simulink model "test_mdl_NI"  (R2018a)
settings: Solver=VariableStepAuto  StartTime=0.0  StopTime=10.0  RelTol=1e-3
(part 2 of 24)

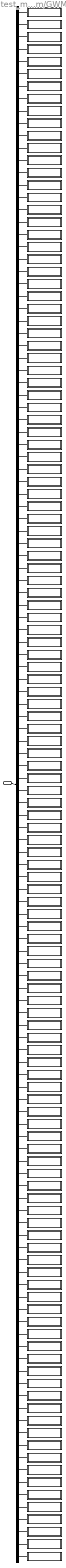
== system test_mdl_NI/Subsystem/GWM ==
  in_port : Inport
  AC_Compressor_Data_FD1_Ox411 : Subsystem
  APIMGPS_Data_Nav_1_FD1_Ox462 : Subsystem
  APIMGPS_Data_Nav_2_FD1_Ox463 : Subsystem
  APIMGPS_Data_Nav_3_FD1_Ox464 : Subsystem
  APIM_Data_FD1_Ox32B : Subsystem
  APIM_Request_Signals_1_FD1_Ox227 : Subsystem
  APIM_Request_Signals_5_FD1_Ox211 : Subsystem
  APIM_Request_Signals_FD1_Ox105 : Subsystem
  APIM_Send_Signals1_FD1_Ox3F1 : Subsystem
  APIM_Send_Signals_2_FD1_Ox215 : Subsystem
  Accel_Data_FD1_Ox92 : Subsystem
  ActiveFrontStrg_Stat2_FD1_Ox8A : Subsystem
  ActiveFrontStrg_Stat_FD1_Ox89 : Subsystem
  Adaptive_Headlamp_Stat_Ox334 : Subsystem
  AllTerrainControlData_FD1_Ox461 : Subsystem
  All_Terrain_Data_FD1_Ox481 : Subsystem
  BCMC_Data_FD1_Ox36F : Subsystem
  BCM_Lamp_Stat_FD1_Ox3C3 : Subsystem
  BattRgenLo_1_FD1_Ox361 : Subsystem
  BattRgenLo_2_FD1_Ox362 : Subsystem
  BattRgenLo_3_FD1_Ox363 : Subsystem
  BattRgenLo_4_FD1_Ox364 : Subsystem
  Battery_Mgmt_24V_FD1_Ox42E : Subsystem
  Battery_Mgmt_2_FD1_Ox42C : Subsystem
  Battery_Mgmt_3_FD1_Ox43C : Subsystem
  Battery_Mgmt_4_FD1_Ox42B : Subsystem
  Battery_Traction_1_FD1_Ox7A : Subsystem
  Battery_Traction_3_FD1_Ox24B : Subsystem
  Battery_Traction_4_FD1_Ox24C : Subsystem
  Battery_Traction_5_FD1_Ox24D : Subsystem
  Battery_Traction_6_FD1_Ox458 : Subsystem
  BodyInfo_3_FD1_Ox3B3 : Subsystem
  Body_Info_10_FD1_Ox3BA : Subsystem
  Body_Info_4_FD1_Ox242 : Subsystem
  Body_Info_6_FD1_Ox38D : Subsystem
  Body_Info_8_FD1_Ox3B9 : Subsystem
  Body_Info_9_FD1_Ox3A3 : Subsystem
  Climate_Cntrl_Data_2_FD1_Ox35E : Subsystem
  Climate_Control_Data_FD1_Ox41A : Subsystem
  Cluster_HEV_Data8_FD1_Ox317 : Subsystem
  Cluster_Info1_FD1_Ox430 : Subsystem
  Cluster_Info_3_FD1_Ox434 : Subsystem
  Cluster_Lighting_Rq_FD1_Ox3C8 : Subsystem
  Compressor_Req_FD1_Ox326 : Subsystem
  CruiseCtrl_Strg_Data_FD1_Ox8B : Subsystem
  DCACA_Data1_FD1_Ox39A : Subsystem
  DCACA_Data2_FD1_Ox39B : Subsystem
  DCACA_Data3_FD1_Ox39C : Subsystem
  DTE_ECGtoHPCM_Ox338 : Subsystem
  Driver_Dr_Stat_FD1_Ox332 : Subsystem
  Dsp_Request_Signals11_FD1_Ox192 : Subsystem
  ECG_Data2_FD1_Ox488 : Subsystem
  ECG_Data3_FD1_Ox375 : Subsystem
  ECG_Data4_FD1_Ox226 : Subsystem
  ECG_Data_FD1_Ox32A : Subsystem
  ElecHorizon_Data1_FD1_Ox22E : Subsystem
  ElecHorizon_Data2_FD1_Ox22F : Subsystem
  FourByFourSwitchData_FD1_Ox460 : Subsystem
  GGCC_Config_Mgmt_ID_1_FD1_Ox40A : Subsystem
  GWM_AutoSar_NetMgmt_FD1_Ox59E : Subsystem
  Gear_Shift_by_Wire_2_FD1_Ox168 : Subsystem
  Gear_Shift_by_Wire_FD1_Ox5A : Subsystem
  GlobalClock_Data_FD1_Ox84 : Subsystem
  Global_PATS_Cntrl_Info_FD1_Ox41 : Subsystem
  Global_PATS_Ctrl_Info2_FD1_Ox42 : Subsystem
  HeadUpDisplayReq_FD1_Ox18B : Subsystem
  IPC_Infotainment_FD1_Ox225 : Subsystem
  IPC_Send_Signals_2_FD1_Ox318 : Subsystem
  LocationServices_3_FD1_Ox21E : Subsystem
  LocationServices_Data1_FD1_Ox47E : Subsystem
  Locking_Systems_2_FD1_Ox331 : Subsystem
  MasterReset_HS3_ECGDat_FD1_Ox233 : Subsystem
  Mc_Send_Signals_2_FD1_Ox2FD : Subsystem
  OTAFuncGWM_ECG_FD1_Ox1B9FFCD8 : Subsystem
  OTAPhysGWM_ECGtoABS_Ox1B90A0D8 : Subsystem
  OTAPhysGWM_ECGtoCCM_Ox1B9054D8 : Subsystem
  OTAPhysGWM_ECGtoIPMA_Ox1B9084D8 : Subsystem
  OTAPhysGWM_ECGtoPCM_Ox1B9040D8 : Subsystem
  OTAPhysGWM_ECGtoSOBDMC_FD1_Ox1B9044D8 : Subsystem
  OTAPhysGWM_ECGtoSODCMC_Ox1B9114D8 : Subsystem
  OTAPhysGWM_ECGtoSODCMD_Ox1B9118D8 : Subsystem
  OTAPhysGWM_ECGtoSODL_Ox1B9188D8 : Subsystem
  OTAPhysGWM_ECGtoSODR_Ox1B918CD8 : Subsystem
  OffBrdChrg_Signals2_Ox27F : Subsystem
  OffBrdChrg_Signals_Ox212 : Subsystem
  PARSEDFuncGWM_ECG_FD1_Ox1BAFFCD8 : Subsystem
  PARSEDPhysGWM_ECGtoABS_Ox1BA0A0D8 : Subsystem
  PARSEDPhysGWM_ECGtoCCM_Ox1BA054D8 : Subsystem
  PARSEDPhysGWM_ECGtoIPMA_Ox1BA084D8 : Subsystem
  PARSEDPhysGWM_ECGtoPCM_Ox1BA040D8 : Subsystem
  PARSEDPhysGWM_ECGtoSODCMC_Ox1BA114D8 : Subsystem
  PARSEDPhysGWM_ECGtoSODCMD_Ox1BA118D8 : Subsystem
  PARSEDPhysGWM_ECGtoSODL_Ox1BA188D8 : Subsystem
  PARSEDPhysGWM_ECGtoSODR_Ox1BA18CD8 : Subsystem
  PARSEDPhysGWMtoSOBDMC_FD1_Ox1BA044D8 : Subsystem
  PARSEDPushFcGWM_ECGtoABS_Ox1BB0A0D8 : Subsystem
  PARSEDPushFcGWM_ECGtoPCM_Ox1BB040D8 : Subsystem
  PHEV_Battery_Data1_FD1_Ox2E4 : Subsystem
  ParkAid_Aud_Warn_CmdM_FD1_Ox30A : Subsystem
  Pass_Dr_Stat_FD1_Ox333 : Subsystem
  Personality_APIM_Data_FD1_Ox3E2 : Subsystem
  Personality_BCM2_Data_FD1_Ox3EB : Subsystem
  Personality_Data_FD1_Ox3E0 : Subsystem
  PowerDistData_2_FD1_Ox36A : Subsystem
  PowerDist_Data1_FD1_Ox390 : Subsystem
  Power_Liftgate_Stat_FD1_Ox313 : Subsystem
  RCMSerialNumber_FD1_Ox454 : Subsystem
  RCMStatusMessage2_FD1_Ox4C : Subsystem
  SmartChargingData_ECG_1_Ox306 : Subsystem
  SmartChargingData_ECG_2_Ox307 : Subsystem
  SmartChargingData_ECG_3_Ox308 : Subsystem
  Steering_Data_FD1_Ox83 : Subsystem
  Steering_Wheel_Data2_FD1_Ox81 : Subsystem
  TCU_Send_Signals_FD1_Ox28B : Subsystem
  TesterPhysicalReqVDM_FD1_Ox721 : Subsystem
  TesterPhysicalResGWM_FD1_Ox71E : Subsystem
  Tire_Pressure_Data_FD1_Ox3B5 : Subsystem
  TrailerAid_Data3_FD1_Ox45C : Subsystem
  TrailerAid_Data_FD1_Ox45A : Subsystem
  TrailerAid_Stat1_FD1_Ox452 : Subsystem
  TrailerAid_Stat2_FD1_Ox457 : Subsystem
  TrailerBrakeInfo_FD1_Ox445 : Subsystem
  TrailerInfo_2_FD1_Ox47A : Subsystem
  TrailerInfo_FD1_Ox443 : Subsystem
  Voltage_Power_Data2_FD1_Ox45F : Subsystem
  Yaw_Data_FD1_Ox91 : Subsystem
  bus_selector : BusSelector  OutputSignals=AC_Compressor_Data_FD1_Ox411,APIMGPS_Data_Nav_1_FD1_Ox462,APIMGPS_Data_Nav_2_FD1_Ox463,APIMGPS_Data_Nav_3_FD1_Ox464,APIM_Data_FD1_Ox32B,APIM_Request_Signals_1_FD1_Ox227,APIM_Request_Signals_5_FD1_Ox211,APIM_Request_Signals_FD1_Ox105,APIM_Send_Signals1_FD1_Ox3F1,APIM_Send_Signals_2_FD1_Ox215,Accel_Data_FD1_Ox92,ActiveFrontStrg_Stat2_FD1_Ox8A,ActiveFrontStrg_Stat_FD1_Ox89,Adaptive_Headlamp_Stat_Ox334,AllTerrainControlData_FD1_Ox461,All_Terrain_Data_FD1_Ox481,BCMC_Data_FD1_Ox36F,BCM_Lamp_Stat_FD1_Ox3C3,BattRgenLo_1_FD1_Ox361,BattRgenLo_2_FD1_Ox362,BattRgenLo_3_FD1_Ox363,BattRgenLo_4_FD1_Ox364,Battery_Mgmt_24V_FD1_Ox42E,Battery_Mgmt_2_FD1_Ox42C,Battery_Mgmt_3_FD1_Ox43C,Battery_Mgmt_4_FD1_Ox42B,Battery_Traction_1_FD1_Ox7A,Battery_Traction_3_FD1_Ox24B,Battery_Traction_4_FD1_Ox24C,Battery_Traction_5_FD1_Ox24D,Battery_Traction_6_FD1_Ox458,BodyInfo_3_FD1_Ox3B3,Body_Info_10_FD1_Ox3BA,Body_Info_4_FD1_Ox242,Body_Info_6_FD1_Ox38D,Body_Info_8_FD1_Ox3B9,Body_Info_9_FD1_Ox3A3,Climate_Cntrl_Data_2_FD1_Ox35E,Climate_Control_Data_FD1_Ox41A,Cluster_HEV_Data8_FD1_Ox317,Cluster_Info1_FD1_Ox430,Cluster_Info_3_FD1_Ox434,Cluster_Lighting_Rq_FD1_Ox3C8,Compressor_Req_FD1_Ox326,CruiseCtrl_Strg_Data_FD1_Ox8B,DCACA_Data1_FD1_Ox39A,DCACA_Data2_FD1_Ox39B,DCACA_Data3_FD1_Ox39C,DTE_ECGtoHPCM_Ox338,Driver_Dr_Stat_FD1_Ox332,Dsp_Request_Signals11_FD1_Ox192,ECG_Data2_FD1_Ox488,ECG_Data3_FD1_Ox375,ECG_Data4_FD1_Ox226,ECG_Data_FD1_Ox32A,ElecHorizon_Data1_FD1_Ox22E,ElecHorizon_Data2_FD1_Ox22F,FourByFourSwitchData_FD1_Ox460,GGCC_Config_Mgmt_ID_1_FD1_Ox40A,GWM_AutoSar_NetMgmt_FD1_Ox59E,Gear_Shift_by_Wire_2_FD1_Ox168,Gear_Shift_by_Wire_FD1_Ox5A,GlobalClock_Data_FD1_Ox84,Global_PATS_Cntrl_Info_FD1_Ox41,Global_PATS_Ctrl_Info2_FD1_Ox42,HeadUpDisplayReq_FD1_Ox18B,IPC_Infotainment_FD1_Ox225,IPC_Send_Signals_2_FD1_Ox318,LocationServices_3_FD1_Ox21E,LocationServices_Data1_FD1_Ox47E,Locking_Systems_2_FD1_Ox331,MasterReset_HS3_ECGDat_FD1_Ox233,Mc_Send_Signals_2_FD1_Ox2FD,OTAFuncGWM_ECG_FD1_Ox1B9FFCD8,OTAPhysGWM_ECGtoABS_Ox1B90A0D8,OTAPhysGWM_ECGtoCCM_Ox1B9054D8,OTAPhysGWM_ECGtoIPMA_Ox1B9084D8,OTAPhysGWM_ECGtoPCM_Ox1B9040D8,OTAPhysGWM_ECGtoSOBDMC_FD1_Ox1B9044D8,OTAPhysGWM_ECGtoSODCMC_Ox1B9114D8,OTAPhysGWM_ECGtoSODCMD_Ox1B9118D8,OTAPhysGWM_ECGtoSODL_Ox1B9188D8,OTAPhysGWM_ECGtoSODR_Ox1B918CD8,OffBrdChrg_Signals_Ox212,OffBrdChrg_Signals2_Ox27F,PARSEDFuncGWM_ECG_FD1_Ox1BAFFCD8,PARSEDPhysGWM_ECGtoABS_Ox1BA0A0D8,PARSEDPhysGWM_ECGtoCCM_Ox1BA054D8,PARSEDPhysGWM_ECGtoIPMA_Ox1BA084D8,PARSEDPhysGWM_ECGtoPCM_Ox1BA040D8,PARSEDPhysGWM_ECGtoSODCMC_Ox1BA114D8,PARSEDPhysGWM_ECGtoSODCMD_Ox1BA118D8,PARSEDPhysGWM_ECGtoSODL_Ox1BA188D8,PARSEDPhysGWM_ECGtoSODR_Ox1BA18CD8,PARSEDPhysGWMtoSOBDMC_FD1_Ox1BA044D8,PARSEDPushFcGWM_ECGtoABS_Ox1BB0A0D8,PARSEDPushFcGWM_ECGtoPCM_Ox1BB040D8,PHEV_Battery_Data1_FD1_Ox2E4,ParkAid_Aud_Warn_CmdM_FD1_Ox30A,Pass_Dr_Stat_FD1_Ox333,Personality_APIM_Data_FD1_Ox3E2,Personality_BCM2_Data_FD1_Ox3EB,Personality_Data_FD1_Ox3E0,PowerDistData_2_FD1_Ox36A,PowerDist_Data1_FD1_Ox390,Power_Liftgate_Stat_FD1_Ox313,RCMSerialNumber_FD1_Ox454,RCMStatusMessage2_FD1_Ox4C,SmartChargingData_ECG_1_Ox306,SmartChargingData_ECG_2_Ox307,SmartChargingData_ECG_3_Ox308,Steering_Data_FD1_Ox83,Steering_Wheel_Data2_FD1_Ox81,TCU_Send_Signals_FD1_Ox28B,TesterPhysicalReqVDM_FD1_Ox721,TesterPhysicalResGWM_FD1_Ox71E,Tire_Pressure_Data_FD1_Ox3B5,TrailerAid_Data3_FD1_Ox45C,TrailerAid_Data_FD1_Ox45A,TrailerAid_Stat1_FD1_Ox452,TrailerAid_Stat2_FD1_Ox457,TrailerBrakeInfo_FD1_Ox445,TrailerInfo_2_FD1_Ox47A,TrailerInfo_FD1_Ox443,Voltage_Power_Data2_FD1_Ox45F,Yaw_Data_FD1_Ox91
  wires:
  in_port/1 -> bus_selector/1  "GWM"
  bus_selector/1 -> AC_Compressor_Data_FD1_Ox411/1(in_port)  "<AC_Compressor_Data_FD1_Ox411>"
  bus_selector/2 -> APIMGPS_Data_Nav_1_FD1_Ox462/1(in_port)  "<APIMGPS_Data_Nav_1_FD1_Ox462>"
  bus_selector/3 -> APIMGPS_Data_Nav_2_FD1_Ox463/1(in_port)  "<APIMGPS_Data_Nav_2_FD1_Ox463>"
  bus_selector/4 -> APIMGPS_Data_Nav_3_FD1_Ox464/1(in_port)  "<APIMGPS_Data_Nav_3_FD1_Ox464>"
  bus_selector/5 -> APIM_Data_FD1_Ox32B/1(in_port)  "<APIM_Data_FD1_Ox32B>"
  bus_selector/6 -> APIM_Request_Signals_1_FD1_Ox227/1(in_port)  "<APIM_Request_Signals_1_FD1_Ox227>"
  bus_selector/7 -> APIM_Request_Signals_5_FD1_Ox211/1(in_port)  "<APIM_Request_Signals_5_FD1_Ox211>"
  bus_selector/8 -> APIM_Request_Signals_FD1_Ox105/1(in_port)  "<APIM_Request_Signals_FD1_Ox105>"
  bus_selector/9 -> APIM_Send_Signals1_FD1_Ox3F1/1(in_port)  "<APIM_Send_Signals1_FD1_Ox3F1>"
  bus_selector/10 -> APIM_Send_Signals_2_FD1_Ox215/1(in_port)  "<APIM_Send_Signals_2_FD1_Ox215>"
  bus_selector/11 -> Accel_Data_FD1_Ox92/1(in_port)  "<Accel_Data_FD1_Ox92>"
  bus_selector/12 -> ActiveFrontStrg_Stat2_FD1_Ox8A/1(in_port)  "<ActiveFrontStrg_Stat2_FD1_Ox8A>"
  bus_selector/13 -> ActiveFrontStrg_Stat_FD1_Ox89/1(in_port)  "<ActiveFrontStrg_Stat_FD1_Ox89>"
  bus_selector/14 -> Adaptive_Headlamp_Stat_Ox334/1(in_port)  "<Adaptive_Headlamp_Stat_Ox334>"
  bus_selector/15 -> AllTerrainControlData_FD1_Ox461/1(in_port)  "<AllTerrainControlData_FD1_Ox461>"
  bus_selector/16 -> All_Terrain_Data_FD1_Ox481/1(in_port)  "<All_Terrain_Data_FD1_Ox481>"
  bus_selector/17 -> BCMC_Data_FD1_Ox36F/1(in_port)  "<BCMC_Data_FD1_Ox36F>"
  bus_selector/18 -> BCM_Lamp_Stat_FD1_Ox3C3/1(in_port)  "<BCM_Lamp_Stat_FD1_Ox3C3>"
  bus_selector/19 -> BattRgenLo_1_FD1_Ox361/1(in_port)  "<BattRgenLo_1_FD1_Ox361>"
  bus_selector/20 -> BattRgenLo_2_FD1_Ox362/1(in_port)  "<BattRgenLo_2_FD1_Ox362>"
  bus_selector/21 -> BattRgenLo_3_FD1_Ox363/1(in_port)  "<BattRgenLo_3_FD1_Ox363>"
  bus_selector/22 -> BattRgenLo_4_FD1_Ox364/1(in_port)  "<BattRgenLo_4_FD1_Ox364>"
  bus_selector/23 -> Battery_Mgmt_24V_FD1_Ox42E/1(in_port)  "<Battery_Mgmt_24V_FD1_Ox42E>"
  bus_selector/24 -> Battery_Mgmt_2_FD1_Ox42C/1(in_port)  "<Battery_Mgmt_2_FD1_Ox42C>"
  bus_selector/25 -> Battery_Mgmt_3_FD1_Ox43C/1(in_port)  "<Battery_Mgmt_3_FD1_Ox43C>"
  bus_selector/26 -> Battery_Mgmt_4_FD1_Ox42B/1(in_port)  "<Battery_Mgmt_4_FD1_Ox42B>"
  bus_selector/27 -> Battery_Traction_1_FD1_Ox7A/1(in_port)  "<Battery_Traction_1_FD1_Ox7A>"
  bus_selector/28 -> Battery_Traction_3_FD1_Ox24B/1(in_port)  "<Battery_Traction_3_FD1_Ox24B>"
  bus_selector/29 -> Battery_Traction_4_FD1_Ox24C/1(in_port)  "<Battery_Traction_4_FD1_Ox24C>"
  bus_selector/30 -> Battery_Traction_5_FD1_Ox24D/1(in_port)  "<Battery_Traction_5_FD1_Ox24D>"
  bus_selector/31 -> Battery_Traction_6_FD1_Ox458/1(in_port)  "<Battery_Traction_6_FD1_Ox458>"
  bus_selector/32 -> BodyInfo_3_FD1_Ox3B3/1(in_port)  "<BodyInfo_3_FD1_Ox3B3>"
  bus_selector/33 -> Body_Info_10_FD1_Ox3BA/1(in_port)  "<Body_Info_10_FD1_Ox3BA>"
  bus_selector/34 -> Body_Info_4_FD1_Ox242/1(in_port)  "<Body_Info_4_FD1_Ox242>"
  bus_selector/35 -> Body_Info_6_FD1_Ox38D/1(in_port)  "<Body_Info_6_FD1_Ox38D>"
  bus_selector/36 -> Body_Info_8_FD1_Ox3B9/1(in_port)  "<Body_Info_8_FD1_Ox3B9>"
  bus_selector/37 -> Body_Info_9_FD1_Ox3A3/1(in_port)  "<Body_Info_9_FD1_Ox3A3>"
  bus_selector/38 -> Climate_Cntrl_Data_2_FD1_Ox35E/1(in_port)  "<Climate_Cntrl_Data_2_FD1_Ox35E>"
  bus_selector/39 -> Climate_Control_Data_FD1_Ox41A/1(in_port)  "<Climate_Control_Data_FD1_Ox41A>"
  bus_selector/40 -> Cluster_HEV_Data8_FD1_Ox317/1(in_port)  "<Cluster_HEV_Data8_FD1_Ox317>"
  bus_selector/41 -> Cluster_Info1_FD1_Ox430/1(in_port)  "<Cluster_Info1_FD1_Ox430>"
  bus_selector/42 -> Cluster_Info_3_FD1_Ox434/1(in_port)  "<Cluster_Info_3_FD1_Ox434>"
  bus_selector/43 -> Cluster_Lighting_Rq_FD1_Ox3C8/1(in_port)  "<Cluster_Lighting_Rq_FD1_Ox3C8>"
  bus_selector/44 -> Compressor_Req_FD1_Ox326/1(in_port)  "<Compressor_Req_FD1_Ox326>"
  bus_selector/45 -> CruiseCtrl_Strg_Data_FD1_Ox8B/1(in_port)  "<CruiseCtrl_Strg_Data_FD1_Ox8B>"
  bus_selector/46 -> DCACA_Data1_FD1_Ox39A/1(in_port)  "<DCACA_Data1_FD1_Ox39A>"
  bus_selector/47 -> DCACA_Data2_FD1_Ox39B/1(in_port)  "<DCACA_Data2_FD1_Ox39B>"
  bus_selector/48 -> DCACA_Data3_FD1_Ox39C/1(in_port)  "<DCACA_Data3_FD1_Ox39C>"
  bus_selector/49 -> DTE_ECGtoHPCM_Ox338/1(in_port)  "<DTE_ECGtoHPCM_Ox338>"
  bus_selector/50 -> Driver_Dr_Stat_FD1_Ox332/1(in_port)  "<Driver_Dr_Stat_FD1_Ox332>"
  bus_selector/51 -> Dsp_Request_Signals11_FD1_Ox192/1(in_port)  "<Dsp_Request_Signals11_FD1_Ox192>"
  bus_selector/52 -> ECG_Data2_FD1_Ox488/1(in_port)  "<ECG_Data2_FD1_Ox488>"
  bus_selector/53 -> ECG_Data3_FD1_Ox375/1(in_port)  "<ECG_Data3_FD1_Ox375>"
  bus_selector/54 -> ECG_Data4_FD1_Ox226/1(in_port)  "<ECG_Data4_FD1_Ox226>"
  bus_selector/55 -> ECG_Data_FD1_Ox32A/1(in_port)  "<ECG_Data_FD1_Ox32A>"
  bus_selector/56 -> ElecHorizon_Data1_FD1_Ox22E/1(in_port)  "<ElecHorizon_Data1_FD1_Ox22E>"
  bus_selector/57 -> ElecHorizon_Data2_FD1_Ox22F/1(in_port)  "<ElecHorizon_Data2_FD1_Ox22F>"
  bus_selector/58 -> FourByFourSwitchData_FD1_Ox460/1(in_port)  "<FourByFourSwitchData_FD1_Ox460>"
  bus_selector/59 -> GGCC_Config_Mgmt_ID_1_FD1_Ox40A/1(in_port)  "<GGCC_Config_Mgmt_ID_1_FD1_Ox40A>"
  bus_selector/60 -> GWM_AutoSar_NetMgmt_FD1_Ox59E/1(in_port)  "<GWM_AutoSar_NetMgmt_FD1_Ox59E>"
  bus_selector/61 -> Gear_Shift_by_Wire_2_FD1_Ox168/1(in_port)  "<Gear_Shift_by_Wire_2_FD1_Ox168>"
  bus_selector/62 -> Gear_Shift_by_Wire_FD1_Ox5A/1(in_port)  "<Gear_Shift_by_Wire_FD1_Ox5A>"
  bus_selector/63 -> GlobalClock_Data_FD1_Ox84/1(in_port)  "<GlobalClock_Data_FD1_Ox84>"
  bus_selector/64 -> Global_PATS_Cntrl_Info_FD1_Ox41/1(in_port)  "<Global_PATS_Cntrl_Info_FD1_Ox41>"
  bus_selector/65 -> Global_PATS_Ctrl_Info2_FD1_Ox42/1(in_port)  "<Global_PATS_Ctrl_Info2_FD1_Ox42>"
  bus_selector/66 -> HeadUpDisplayReq_FD1_Ox18B/1(in_port)  "<HeadUpDisplayReq_FD1_Ox18B>"
  bus_selector/67 -> IPC_Infotainment_FD1_Ox225/1(in_port)  "<IPC_Infotainment_FD1_Ox225>"
  bus_selector/68 -> IPC_Send_Signals_2_FD1_Ox318/1(in_port)  "<IPC_Send_Signals_2_FD1_Ox318>"
  bus_selector/69 -> LocationServices_3_FD1_Ox21E/1(in_port)  "<LocationServices_3_FD1_Ox21E>"
  bus_selector/70 -> LocationServices_Data1_FD1_Ox47E/1(in_port)  "<LocationServices_Data1_FD1_Ox47E>"
  bus_selector/71 -> Locking_Systems_2_FD1_Ox331/1(in_port)  "<Locking_Systems_2_FD1_Ox331>"
  bus_selector/72 -> MasterReset_HS3_ECGDat_FD1_Ox233/1(in_port)  "<MasterReset_HS3_ECGDat_FD1_Ox233>"
  bus_selector/73 -> Mc_Send_Signals_2_FD1_Ox2FD/1(in_port)  "<Mc_Send_Signals_2_FD1_Ox2FD>"
  bus_selector/74 -> OTAFuncGWM_ECG_FD1_Ox1B9FFCD8/1(in_port)  "<OTAFuncGWM_ECG_FD1_Ox1B9FFCD8>"
  bus_selector/75 -> OTAPhysGWM_ECGtoABS_Ox1B90A0D8/1(in_port)  "<OTAPhysGWM_ECGtoABS_Ox1B90A0D8>"
  bus_selector/76 -> OTAPhysGWM_ECGtoCCM_Ox1B9054D8/1(in_port)  "<OTAPhysGWM_ECGtoCCM_Ox1B9054D8>"
  bus_selector/77 -> OTAPhysGWM_ECGtoIPMA_Ox1B9084D8/1(in_port)  "<OTAPhysGWM_ECGtoIPMA_Ox1B9084D8>"
  bus_selector/78 -> OTAPhysGWM_ECGtoPCM_Ox1B9040D8/1(in_port)  "<OTAPhysGWM_ECGtoPCM_Ox1B9040D8>"
  bus_selector/79 -> OTAPhysGWM_ECGtoSOBDMC_FD1_Ox1B9044D8/1(in_port)  "<OTAPhysGWM_ECGtoSOBDMC_FD1_Ox1B9044D8>"
  bus_selector/80 -> OTAPhysGWM_ECGtoSODCMC_Ox1B9114D8/1(in_port)  "<OTAPhysGWM_ECGtoSODCMC_Ox1B9114D8>"
  bus_selector/81 -> OTAPhysGWM_ECGtoSODCMD_Ox1B9118D8/1(in_port)  "<OTAPhysGWM_ECGtoSODCMD_Ox1B9118D8>"
  bus_selector/82 -> OTAPhysGWM_ECGtoSODL_Ox1B9188D8/1(in_port)  "<OTAPhysGWM_ECGtoSODL_Ox1B9188D8>"
  bus_selector/83 -> OTAPhysGWM_ECGtoSODR_Ox1B918CD8/1(in_port)  "<OTAPhysGWM_ECGtoSODR_Ox1B918CD8>"
  bus_selector/84 -> OffBrdChrg_Signals_Ox212/1(in_port)  "<OffBrdChrg_Signals_Ox212>"
  bus_selector/85 -> OffBrdChrg_Signals2_Ox27F/1(in_port)  "<OffBrdChrg_Signals2_Ox27F>"
  bus_selector/86 -> PARSEDFuncGWM_ECG_FD1_Ox1BAFFCD8/1(in_port)  "<PARSEDFuncGWM_ECG_FD1_Ox1BAFFCD8>"
  bus_selector/87 -> PARSEDPhysGWM_ECGtoABS_Ox1BA0A0D8/1(in_port)  "<PARSEDPhysGWM_ECGtoABS_Ox1BA0A0D8>"
  bus_selector/88 -> PARSEDPhysGWM_ECGtoCCM_Ox1BA054D8/1(in_port)  "<PARSEDPhysGWM_ECGtoCCM_Ox1BA054D8>"
  bus_selector/89 -> PARSEDPhysGWM_ECGtoIPMA_Ox1BA084D8/1(in_port)  "<PARSEDPhysGWM_ECGtoIPMA_Ox1BA084D8>"
  bus_selector/90 -> PARSEDPhysGWM_ECGtoPCM_Ox1BA040D8/1(in_port)  "<PARSEDPhysGWM_ECGtoPCM_Ox1BA040D8>"
  bus_selector/91 -> PARSEDPhysGWM_ECGtoSODCMC_Ox1BA114D8/1(in_port)  "<PARSEDPhysGWM_ECGtoSODCMC_Ox1BA114D8>"
  bus_selector/92 -> PARSEDPhysGWM_ECGtoSODCMD_Ox1BA118D8/1(in_port)  "<PARSEDPhysGWM_ECGtoSODCMD_Ox1BA118D8>"
  bus_selector/93 -> PARSEDPhysGWM_ECGtoSODL_Ox1BA188D8/1(in_port)  "<PARSEDPhysGWM_ECGtoSODL_Ox1BA188D8>"
  bus_selector/94 -> PARSEDPhysGWM_ECGtoSODR_Ox1BA18CD8/1(in_port)  "<PARSEDPhysGWM_ECGtoSODR_Ox1BA18CD8>"
  bus_selector/95 -> PARSEDPhysGWMtoSOBDMC_FD1_Ox1BA044D8/1(in_port)  "<PARSEDPhysGWMtoSOBDMC_FD1_Ox1BA044D8>"
  bus_selector/96 -> PARSEDPushFcGWM_ECGtoABS_Ox1BB0A0D8/1(in_port)  "<PARSEDPushFcGWM_ECGtoABS_Ox1BB0A0D8>"
  bus_selector/97 -> PARSEDPushFcGWM_ECGtoPCM_Ox1BB040D8/1(in_port)  "<PARSEDPushFcGWM_ECGtoPCM_Ox1BB040D8>"
  bus_selector/98 -> PHEV_Battery_Data1_FD1_Ox2E4/1(in_port)  "<PHEV_Battery_Data1_FD1_Ox2E4>"
  bus_selector/99 -> ParkAid_Aud_Warn_CmdM_FD1_Ox30A/1(in_port)  "<ParkAid_Aud_Warn_CmdM_FD1_Ox30A>"
  bus_selector/100 -> Pass_Dr_Stat_FD1_Ox333/1(in_port)  "<Pass_Dr_Stat_FD1_Ox333>"
  bus_selector/101 -> Personality_APIM_Data_FD1_Ox3E2/1(in_port)  "<Personality_APIM_Data_FD1_Ox3E2>"
  bus_selector/102 -> Personality_BCM2_Data_FD1_Ox3EB/1(in_port)  "<Personality_BCM2_Data_FD1_Ox3EB>"
  bus_selector/103 -> Personality_Data_FD1_Ox3E0/1(in_port)  "<Personality_Data_FD1_Ox3E0>"
  bus_selector/104 -> PowerDistData_2_FD1_Ox36A/1(in_port)  "<PowerDistData_2_FD1_Ox36A>"
  bus_selector/105 -> PowerDist_Data1_FD1_Ox390/1(in_port)  "<PowerDist_Data1_FD1_Ox390>"
  bus_selector/106 -> Power_Liftgate_Stat_FD1_Ox313/1(in_port)  "<Power_Liftgate_Stat_FD1_Ox313>"
  bus_selector/107 -> RCMSerialNumber_FD1_Ox454/1(in_port)  "<RCMSerialNumber_FD1_Ox454>"
  bus_selector/108 -> RCMStatusMessage2_FD1_Ox4C/1(in_port)  "<RCMStatusMessage2_FD1_Ox4C>"
  bus_selector/109 -> SmartChargingData_ECG_1_Ox306/1(in_port)  "<SmartChargingData_ECG_1_Ox306>"
  bus_selector/110 -> SmartChargingData_ECG_2_Ox307/1(in_port)  "<SmartChargingData_ECG_2_Ox307>"
  bus_selector/111 -> SmartChargingData_ECG_3_Ox308/1(in_port)  "<SmartChargingData_ECG_3_Ox308>"
  bus_selector/112 -> Steering_Data_FD1_Ox83/1(in_port)  "<Steering_Data_FD1_Ox83>"
  bus_selector/113 -> Steering_Wheel_Data2_FD1_Ox81/1(in_port)  "<Steering_Wheel_Data2_FD1_Ox81>"
  bus_selector/114 -> TCU_Send_Signals_FD1_Ox28B/1(in_port)  "<TCU_Send_Signals_FD1_Ox28B>"
  bus_selector/115 -> TesterPhysicalReqVDM_FD1_Ox721/1(in_port)  "<TesterPhysicalReqVDM_FD1_Ox721>"
  bus_selector/116 -> TesterPhysicalResGWM_FD1_Ox71E/1(in_port)  "<TesterPhysicalResGWM_FD1_Ox71E>"
  bus_selector/117 -> Tire_Pressure_Data_FD1_Ox3B5/1(in_port)  "<Tire_Pressure_Data_FD1_Ox3B5>"
  bus_selector/118 -> TrailerAid_Data3_FD1_Ox45C/1(in_port)  "<TrailerAid_Data3_FD1_Ox45C>"
  bus_selector/119 -> TrailerAid_Data_FD1_Ox45A/1(in_port)  "<TrailerAid_Data_FD1_Ox45A>"
  bus_selector/120 -> TrailerAid_Stat1_FD1_Ox452/1(in_port)  "<TrailerAid_Stat1_FD1_Ox452>"
  bus_selector/121 -> TrailerAid_Stat2_FD1_Ox457/1(in_port)  "<TrailerAid_Stat2_FD1_Ox457>"
  bus_selector/122 -> TrailerBrakeInfo_FD1_Ox445/1(in_port)  "<TrailerBrakeInfo_FD1_Ox445>"
  bus_selector/123 -> TrailerInfo_2_FD1_Ox47A/1(in_port)  "<TrailerInfo_2_FD1_Ox47A>"
  bus_selector/124 -> TrailerInfo_FD1_Ox443/1(in_port)  "<TrailerInfo_FD1_Ox443>"
  bus_selector/125 -> Voltage_Power_Data2_FD1_Ox45F/1(in_port)  "<Voltage_Power_Data2_FD1_Ox45F>"
  bus_selector/126 -> Yaw_Data_FD1_Ox91/1(in_port)  "<Yaw_Data_FD1_Ox91>"

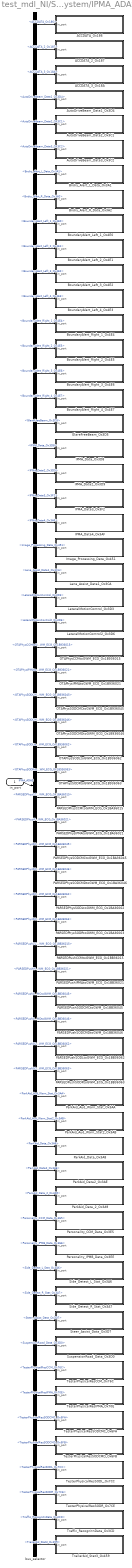
== system test_mdl_NI/Subsystem/IPMA_ADAS ==
  in_port : Inport
  ACCDATA_2_Ox187 : Subsystem
  ACCDATA_3_Ox18A : Subsystem
  ACCDATA_Ox186 : Subsystem
  AutoDriveBeam_Data1_Ox3D4 : Subsystem
  AutoDriveBeam_Data2_Ox3C1 : Subsystem
  AutoDriveBeam_Data3_Ox3C2 : Subsystem
  Bndry_Alert_L_Data_Ox3A1 : Subsystem
  Bndry_Alert_R_Data_Ox3A2 : Subsystem
  BoundaryAlert_Left_1_Ox4E0 : Subsystem
  BoundaryAlert_Left_2_Ox4E1 : Subsystem
  BoundaryAlert_Left_3_Ox4E2 : Subsystem
  BoundaryAlert_Left_4_Ox4E3 : Subsystem
  BoundaryAlert_Right_1_Ox4E4 : Subsystem
  BoundaryAlert_Right_2_Ox4E5 : Subsystem
  BoundaryAlert_Right_3_Ox4E6 : Subsystem
  BoundaryAlert_Right_4_Ox4E7 : Subsystem
  GlareFreeBeam_Ox3D5 : Subsystem
  IPMA_Data2_Ox3D9 : Subsystem
  IPMA_Data3_Ox3F2 : Subsystem
  IPMA_Data4_Ox3AF : Subsystem
  IPMA_Data_Ox3D8 : Subsystem
  Image_Processing_Data_Ox451 : Subsystem
  Lane_Assist_Data1_Ox3CA : Subsystem
  LateralMotionControl2_Ox3D6 : Subsystem
  LateralMotionControl_Ox3D3 : Subsystem
  OTAPhysCCMtoGWM_ECG_Ox1B936015 : Subsystem
  OTAPhysIPMAtoGWM_ECG_Ox1B936021 : Subsystem
  OTAPhysSODCMCtoGWM_ECG_Ox1B936045 : Subsystem
  OTAPhysSODCMDtoGWM_ECG_Ox1B936046 : Subsystem
  OTAPhysSODLtoGWM_ECG_Ox1B936062 : Subsystem
  OTAPhysSODRtoGWM_ECG_Ox1B936063 : Subsystem
  PARSEDPhysCCMtoGWM_ECG_Ox1BA36015 : Subsystem
  PARSEDPhysIPMAtoGWM_ECG_Ox1BA36021 : Subsystem
  PARSEDPhysSODCMCtoGWM_ECG_Ox1BA36045 : Subsystem
  PARSEDPhysSODCMDtoGWM_ECG_Ox1BA36046 : Subsystem
  PARSEDPhysSODLtoGWM_ECG_Ox1BA36062 : Subsystem
  PARSEDPhysSODRtoGWM_ECG_Ox1BA36063 : Subsystem
  PARSEDPushCCMtoGWM_ECG_Ox1BB36015 : Subsystem
  PARSEDPushIPMAtoGWM_ECG_Ox1BB36021 : Subsystem
  PARSEDPushSODCMCtoGWM_Ox1BB36045 : Subsystem
  PARSEDPushSODCMDtoGWM_Ox1BB36046 : Subsystem
  PARSEDPushSODLtoGWM_ECG_Ox1BB36062 : Subsystem
  PARSEDPushSODRtoGWM_ECG_Ox1BB36063 : Subsystem
  ParkAid_Aud_Warn_Stat2_Ox3AB : Subsystem
  ParkAid_Aud_Warn_Stat_Ox3AA : Subsystem
  ParkAid_Data2_Ox3AE : Subsystem
  ParkAid_Data_2_Ox3A9 : Subsystem
  ParkAid_Data_Ox3A8 : Subsystem
  Personality_CCM_Data_Ox3E5 : Subsystem
  Personality_IPMB_Data_Ox3EE : Subsystem
  Side_Detect_L_Stat_Ox3A6 : Subsystem
  Side_Detect_R_Stat_Ox3A7 : Subsystem
  Steer_Assist_Data_Ox3D7 : Subsystem
  SuspensionRoad_Data_Ox3D0 : Subsystem
  TesterPhysicalResCCM_Ox76C : Subsystem
  TesterPhysicalResIPMA_Ox70E : Subsystem
  TesterPhysicalResSODCMC_Ox6FA : Subsystem
  TesterPhysicalResSODCMD_Ox6FB : Subsystem
  TesterPhysicalResSODL_Ox7CC : Subsystem
  TesterPhysicalResSODR_Ox7CE : Subsystem
  Traffic_RecognitnData_Ox3CD : Subsystem
  TrailerAid_Stat3_Ox459 : Subsystem
  bus_selector : BusSelector  OutputSignals=ACCDATA_Ox186,ACCDATA_2_Ox187,ACCDATA_3_Ox18A,AutoDriveBeam_Data1_Ox3D4,AutoDriveBeam_Data2_Ox3C1,AutoDriveBeam_Data3_Ox3C2,Bndry_Alert_L_Data_Ox3A1,Bndry_Alert_R_Data_Ox3A2,BoundaryAlert_Left_1_Ox4E0,BoundaryAlert_Left_2_Ox4E1,BoundaryAlert_Left_3_Ox4E2,BoundaryAlert_Left_4_Ox4E3,BoundaryAlert_Right_1_Ox4E4,BoundaryAlert_Right_2_Ox4E5,BoundaryAlert_Right_3_Ox4E6,BoundaryAlert_Right_4_Ox4E7,GlareFreeBeam_Ox3D5,IPMA_Data_Ox3D8,IPMA_Data2_Ox3D9,IPMA_Data3_Ox3F2,IPMA_Data4_Ox3AF,Image_Processing_Data_Ox451,Lane_Assist_Data1_Ox3CA,LateralMotionControl_Ox3D3,LateralMotionControl2_Ox3D6,OTAPhysCCMtoGWM_ECG_Ox1B936015,OTAPhysIPMAtoGWM_ECG_Ox1B936021,OTAPhysSODCMCtoGWM_ECG_Ox1B936045,OTAPhysSODCMDtoGWM_ECG_Ox1B936046,OTAPhysSODLtoGWM_ECG_Ox1B936062,OTAPhysSODRtoGWM_ECG_Ox1B936063,PARSEDPhysCCMtoGWM_ECG_Ox1BA36015,PARSEDPhysIPMAtoGWM_ECG_Ox1BA36021,PARSEDPhysSODCMCtoGWM_ECG_Ox1BA36045,PARSEDPhysSODCMDtoGWM_ECG_Ox1BA36046,PARSEDPhysSODLtoGWM_ECG_Ox1BA36062,PARSEDPhysSODRtoGWM_ECG_Ox1BA36063,PARSEDPushCCMtoGWM_ECG_Ox1BB36015,PARSEDPushIPMAtoGWM_ECG_Ox1BB36021,PARSEDPushSODCMCtoGWM_Ox1BB36045,PARSEDPushSODCMDtoGWM_Ox1BB36046,PARSEDPushSODLtoGWM_ECG_Ox1BB36062,PARSEDPushSODRtoGWM_ECG_Ox1BB36063,ParkAid_Aud_Warn_Stat_Ox3AA,ParkAid_Aud_Warn_Stat2_Ox3AB,ParkAid_Data_Ox3A8,ParkAid_Data2_Ox3AE,ParkAid_Data_2_Ox3A9,Personality_CCM_Data_Ox3E5,Personality_IPMB_Data_Ox3EE,Side_Detect_L_Stat_Ox3A6,Side_Detect_R_Stat_Ox3A7,Steer_Assist_Data_Ox3D7,SuspensionRoad_Data_Ox3D0,TesterPhysicalResCCM_Ox76C,TesterPhysicalResIPMA_Ox70E,TesterPhysicalResSODCMC_Ox6FA,TesterPhysicalResSODCMD_Ox6FB,TesterPhysicalResSODL_Ox7CC,TesterPhysicalResSODR_Ox7CE,Traffic_RecognitnData_Ox3CD,TrailerAid_Stat3_Ox459
  wires:
  in_port/1 -> bus_selector/1  "IPMA_ADAS"
  bus_selector/1 -> ACCDATA_Ox186/1(in_port)  "<ACCDATA_Ox186>"
  bus_selector/2 -> ACCDATA_2_Ox187/1(in_port)  "<ACCDATA_2_Ox187>"
  bus_selector/3 -> ACCDATA_3_Ox18A/1(in_port)  "<ACCDATA_3_Ox18A>"
  bus_selector/4 -> AutoDriveBeam_Data1_Ox3D4/1(in_port)  "<AutoDriveBeam_Data1_Ox3D4>"
  bus_selector/5 -> AutoDriveBeam_Data2_Ox3C1/1(in_port)  "<AutoDriveBeam_Data2_Ox3C1>"
  bus_selector/6 -> AutoDriveBeam_Data3_Ox3C2/1(in_port)  "<AutoDriveBeam_Data3_Ox3C2>"
  bus_selector/7 -> Bndry_Alert_L_Data_Ox3A1/1(in_port)  "<Bndry_Alert_L_Data_Ox3A1>"
  bus_selector/8 -> Bndry_Alert_R_Data_Ox3A2/1(in_port)  "<Bndry_Alert_R_Data_Ox3A2>"
  bus_selector/9 -> BoundaryAlert_Left_1_Ox4E0/1(in_port)  "<BoundaryAlert_Left_1_Ox4E0>"
  bus_selector/10 -> BoundaryAlert_Left_2_Ox4E1/1(in_port)  "<BoundaryAlert_Left_2_Ox4E1>"
  bus_selector/11 -> BoundaryAlert_Left_3_Ox4E2/1(in_port)  "<BoundaryAlert_Left_3_Ox4E2>"
  bus_selector/12 -> BoundaryAlert_Left_4_Ox4E3/1(in_port)  "<BoundaryAlert_Left_4_Ox4E3>"
  bus_selector/13 -> BoundaryAlert_Right_1_Ox4E4/1(in_port)  "<BoundaryAlert_Right_1_Ox4E4>"
  bus_selector/14 -> BoundaryAlert_Right_2_Ox4E5/1(in_port)  "<BoundaryAlert_Right_2_Ox4E5>"
  bus_selector/15 -> BoundaryAlert_Right_3_Ox4E6/1(in_port)  "<BoundaryAlert_Right_3_Ox4E6>"
  bus_selector/16 -> BoundaryAlert_Right_4_Ox4E7/1(in_port)  "<BoundaryAlert_Right_4_Ox4E7>"
  bus_selector/17 -> GlareFreeBeam_Ox3D5/1(in_port)  "<GlareFreeBeam_Ox3D5>"
  bus_selector/18 -> IPMA_Data_Ox3D8/1(in_port)  "<IPMA_Data_Ox3D8>"
  bus_selector/19 -> IPMA_Data2_Ox3D9/1(in_port)  "<IPMA_Data2_Ox3D9>"
  bus_selector/20 -> IPMA_Data3_Ox3F2/1(in_port)  "<IPMA_Data3_Ox3F2>"
  bus_selector/21 -> IPMA_Data4_Ox3AF/1(in_port)  "<IPMA_Data4_Ox3AF>"
  bus_selector/22 -> Image_Processing_Data_Ox451/1(in_port)  "<Image_Processing_Data_Ox451>"
  bus_selector/23 -> Lane_Assist_Data1_Ox3CA/1(in_port)  "<Lane_Assist_Data1_Ox3CA>"
  bus_selector/24 -> LateralMotionControl_Ox3D3/1(in_port)  "<LateralMotionControl_Ox3D3>"
  bus_selector/25 -> LateralMotionControl2_Ox3D6/1(in_port)  "<LateralMotionControl2_Ox3D6>"
  bus_selector/26 -> OTAPhysCCMtoGWM_ECG_Ox1B936015/1(in_port)  "<OTAPhysCCMtoGWM_ECG_Ox1B936015>"
  bus_selector/27 -> OTAPhysIPMAtoGWM_ECG_Ox1B936021/1(in_port)  "<OTAPhysIPMAtoGWM_ECG_Ox1B936021>"
  bus_selector/28 -> OTAPhysSODCMCtoGWM_ECG_Ox1B936045/1(in_port)  "<OTAPhysSODCMCtoGWM_ECG_Ox1B936045>"
  bus_selector/29 -> OTAPhysSODCMDtoGWM_ECG_Ox1B936046/1(in_port)  "<OTAPhysSODCMDtoGWM_ECG_Ox1B936046>"
  bus_selector/30 -> OTAPhysSODLtoGWM_ECG_Ox1B936062/1(in_port)  "<OTAPhysSODLtoGWM_ECG_Ox1B936062>"
  bus_selector/31 -> OTAPhysSODRtoGWM_ECG_Ox1B936063/1(in_port)  "<OTAPhysSODRtoGWM_ECG_Ox1B936063>"
  bus_selector/32 -> PARSEDPhysCCMtoGWM_ECG_Ox1BA36015/1(in_port)  "<PARSEDPhysCCMtoGWM_ECG_Ox1BA36015>"
  bus_selector/33 -> PARSEDPhysIPMAtoGWM_ECG_Ox1BA36021/1(in_port)  "<PARSEDPhysIPMAtoGWM_ECG_Ox1BA36021>"
  bus_selector/34 -> PARSEDPhysSODCMCtoGWM_ECG_Ox1BA36045/1(in_port)  "<PARSEDPhysSODCMCtoGWM_ECG_Ox1BA36045>"
  bus_selector/35 -> PARSEDPhysSODCMDtoGWM_ECG_Ox1BA36046/1(in_port)  "<PARSEDPhysSODCMDtoGWM_ECG_Ox1BA36046>"
  bus_selector/36 -> PARSEDPhysSODLtoGWM_ECG_Ox1BA36062/1(in_port)  "<PARSEDPhysSODLtoGWM_ECG_Ox1BA36062>"
  bus_selector/37 -> PARSEDPhysSODRtoGWM_ECG_Ox1BA36063/1(in_port)  "<PARSEDPhysSODRtoGWM_ECG_Ox1BA36063>"
  bus_selector/38 -> PARSEDPushCCMtoGWM_ECG_Ox1BB36015/1(in_port)  "<PARSEDPushCCMtoGWM_ECG_Ox1BB36015>"
  bus_selector/39 -> PARSEDPushIPMAtoGWM_ECG_Ox1BB36021/1(in_port)  "<PARSEDPushIPMAtoGWM_ECG_Ox1BB36021>"
  bus_selector/40 -> PARSEDPushSODCMCtoGWM_Ox1BB36045/1(in_port)  "<PARSEDPushSODCMCtoGWM_Ox1BB36045>"
  bus_selector/41 -> PARSEDPushSODCMDtoGWM_Ox1BB36046/1(in_port)  "<PARSEDPushSODCMDtoGWM_Ox1BB36046>"
  bus_selector/42 -> PARSEDPushSODLtoGWM_ECG_Ox1BB36062/1(in_port)  "<PARSEDPushSODLtoGWM_ECG_Ox1BB36062>"
  bus_selector/43 -> PARSEDPushSODRtoGWM_ECG_Ox1BB36063/1(in_port)  "<PARSEDPushSODRtoGWM_ECG_Ox1BB36063>"
  bus_selector/44 -> ParkAid_Aud_Warn_Stat_Ox3AA/1(in_port)  "<ParkAid_Aud_Warn_Stat_Ox3AA>"
  bus_selector/45 -> ParkAid_Aud_Warn_Stat2_Ox3AB/1(in_port)  "<ParkAid_Aud_Warn_Stat2_Ox3AB>"
  bus_selector/46 -> ParkAid_Data_Ox3A8/1(in_port)  "<ParkAid_Data_Ox3A8>"
  bus_selector/47 -> ParkAid_Data2_Ox3AE/1(in_port)  "<ParkAid_Data2_Ox3AE>"
  bus_selector/48 -> ParkAid_Data_2_Ox3A9/1(in_port)  "<ParkAid_Data_2_Ox3A9>"
  bus_selector/49 -> Personality_CCM_Data_Ox3E5/1(in_port)  "<Personality_CCM_Data_Ox3E5>"
  bus_selector/50 -> Personality_IPMB_Data_Ox3EE/1(in_port)  "<Personality_IPMB_Data_Ox3EE>"
  bus_selector/51 -> Side_Detect_L_Stat_Ox3A6/1(in_port)  "<Side_Detect_L_Stat_Ox3A6>"
  bus_selector/52 -> Side_Detect_R_Stat_Ox3A7/1(in_port)  "<Side_Detect_R_Stat_Ox3A7>"
  bus_selector/53 -> Steer_Assist_Data_Ox3D7/1(in_port)  "<Steer_Assist_Data_Ox3D7>"
  bus_selector/54 -> SuspensionRoad_Data_Ox3D0/1(in_port)  "<SuspensionRoad_Data_Ox3D0>"
  bus_selector/55 -> TesterPhysicalResCCM_Ox76C/1(in_port)  "<TesterPhysicalResCCM_Ox76C>"
  bus_selector/56 -> TesterPhysicalResIPMA_Ox70E/1(in_port)  "<TesterPhysicalResIPMA_Ox70E>"
  bus_selector/57 -> TesterPhysicalResSODCMC_Ox6FA/1(in_port)  "<TesterPhysicalResSODCMC_Ox6FA>"
  bus_selector/58 -> TesterPhysicalResSODCMD_Ox6FB/1(in_port)  "<TesterPhysicalResSODCMD_Ox6FB>"
  bus_selector/59 -> TesterPhysicalResSODL_Ox7CC/1(in_port)  "<TesterPhysicalResSODL_Ox7CC>"
  bus_selector/60 -> TesterPhysicalResSODR_Ox7CE/1(in_port)  "<TesterPhysicalResSODR_Ox7CE>"
  bus_selector/61 -> Traffic_RecognitnData_Ox3CD/1(in_port)  "<Traffic_RecognitnData_Ox3CD>"
  bus_selector/62 -> TrailerAid_Stat3_Ox459/1(in_port)  "<TrailerAid_Stat3_Ox459>"

== system test_mdl_NI/Subsystem/PCM ==
  in_port : Inport
  DCACA_Data4_Ox36E : Subsystem
  EngBrakeData_Ox165 : Subsystem
  EngVehicleSpThrottle2_Ox202 : Subsystem
  EngVehicleSpThrottle_Ox204 : Subsystem
  EngineClimateData_Ox178 : Subsystem
  EngineData_16_Ox17C : Subsystem
  EngineData_1_Ox171 : Subsystem
  EngineData_6_Ox156 : Subsystem
  EngineData_7_Ox179 : Subsystem
  Engine_Clutch_Data_Ox42F : Subsystem
  Gear_Shift_by_Wire_3_Ox5C : Subsystem
  Global_PATS_TargetInfo_Ox47 : Subsystem
  Low_Voltage_Power_Data_FD1_Ox43D : Subsystem
  OTAPhysPCMtoGWM_ECG_Ox1B936010 : Subsystem
  PARSEDPhysPCMtoGWM_ECG_Ox1BA36010 : Subsystem
  PARSEDPushPCMtoGWM_ECG_Ox1BB36010 : Subsystem
  PCM_AutoSar_NetworkMgmt_Ox595 : Subsystem
  PCM_Rapid_Data_Response_1_Ox6A0 : Subsystem
  PCM_Rapid_Data_Response_2_Ox6A1 : Subsystem
  PowertrainData_10_Ox176 : Subsystem
  PowertrainData_1_Ox421 : Subsystem
  PowertrainData_2_Ox42D : Subsystem
  PowertrainData_3_Ox43E : Subsystem
  PowertrainData_6_Ox205 : Subsystem
  PowertrainData_7_Ox41F : Subsystem
  PowertrainData_9_Ox44C : Subsystem
  Powertrain_Data_4_Ox424 : Subsystem
  Powertrain_Data_5_Ox43F : Subsystem
  Stop_Start_Ox166 : Subsystem
  TesterPhysicalResPCM_Ox7E8 : Subsystem
  TorqueDataEngFlags_Ox200 : Subsystem
  TransGearData_Ox230 : Subsystem
  VehicleOperatingModes_Ox167 : Subsystem
  bus_selector : BusSelector  OutputSignals=DCACA_Data4_Ox36E,EngBrakeData_Ox165,EngVehicleSpThrottle_Ox204,EngVehicleSpThrottle2_Ox202,EngineClimateData_Ox178,EngineData_1_Ox171,EngineData_16_Ox17C,EngineData_6_Ox156,EngineData_7_Ox179,Engine_Clutch_Data_Ox42F,Gear_Shift_by_Wire_3_Ox5C,Global_PATS_TargetInfo_Ox47,Low_Voltage_Power_Data_FD1_Ox43D,OTAPhysPCMtoGWM_ECG_Ox1B936010,PARSEDPhysPCMtoGWM_ECG_Ox1BA36010,PARSEDPushPCMtoGWM_ECG_Ox1BB36010,PCM_AutoSar_NetworkMgmt_Ox595,PCM_Rapid_Data_Response_1_Ox6A0,PCM_Rapid_Data_Response_2_Ox6A1,PowertrainData_1_Ox421,PowertrainData_10_Ox176,PowertrainData_2_Ox42D,PowertrainData_3_Ox43E,PowertrainData_6_Ox205,PowertrainData_7_Ox41F,PowertrainData_9_Ox44C,Powertrain_Data_4_Ox424,Powertrain_Data_5_Ox43F,Stop_Start_Ox166,TesterPhysicalResPCM_Ox7E8,TorqueDataEngFlags_Ox200,TransGearData_Ox230,VehicleOperatingModes_Ox167
  wires:
  in_port/1 -> bus_selector/1  "PCM"
  bus_selector/1 -> DCACA_Data4_Ox36E/1(in_port)  "<DCACA_Data4_Ox36E>"
  bus_selector/2 -> EngBrakeData_Ox165/1(in_port)  "<EngBrakeData_Ox165>"
  bus_selector/3 -> EngVehicleSpThrottle_Ox204/1(in_port)  "<EngVehicleSpThrottle_Ox204>"
  bus_selector/4 -> EngVehicleSpThrottle2_Ox202/1(in_port)  "<EngVehicleSpThrottle2_Ox202>"
  bus_selector/5 -> EngineClimateData_Ox178/1(in_port)  "<EngineClimateData_Ox178>"
  bus_selector/6 -> EngineData_1_Ox171/1(in_port)  "<EngineData_1_Ox171>"
  bus_selector/7 -> EngineData_16_Ox17C/1(in_port)  "<EngineData_16_Ox17C>"
  bus_selector/8 -> EngineData_6_Ox156/1(in_port)  "<EngineData_6_Ox156>"
  bus_selector/9 -> EngineData_7_Ox179/1(in_port)  "<EngineData_7_Ox179>"
  bus_selector/10 -> Engine_Clutch_Data_Ox42F/1(in_port)  "<Engine_Clutch_Data_Ox42F>"
  bus_selector/11 -> Gear_Shift_by_Wire_3_Ox5C/1(in_port)  "<Gear_Shift_by_Wire_3_Ox5C>"
  bus_selector/12 -> Global_PATS_TargetInfo_Ox47/1(in_port)  "<Global_PATS_TargetInfo_Ox47>"
  bus_selector/13 -> Low_Voltage_Power_Data_FD1_Ox43D/1(in_port)  "<Low_Voltage_Power_Data_FD1_Ox43D>"
  bus_selector/14 -> OTAPhysPCMtoGWM_ECG_Ox1B936010/1(in_port)  "<OTAPhysPCMtoGWM_ECG_Ox1B936010>"
  bus_selector/15 -> PARSEDPhysPCMtoGWM_ECG_Ox1BA36010/1(in_port)  "<PARSEDPhysPCMtoGWM_ECG_Ox1BA36010>"
  bus_selector/16 -> PARSEDPushPCMtoGWM_ECG_Ox1BB36010/1(in_port)  "<PARSEDPushPCMtoGWM_ECG_Ox1BB36010>"
  bus_selector/17 -> PCM_AutoSar_NetworkMgmt_Ox595/1(in_port)  "<PCM_AutoSar_NetworkMgmt_Ox595>"
  bus_selector/18 -> PCM_Rapid_Data_Response_1_Ox6A0/1(in_port)  "<PCM_Rapid_Data_Response_1_Ox6A0>"
  bus_selector/19 -> PCM_Rapid_Data_Response_2_Ox6A1/1(in_port)  "<PCM_Rapid_Data_Response_2_Ox6A1>"
  bus_selector/20 -> PowertrainData_1_Ox421/1(in_port)  "<PowertrainData_1_Ox421>"
  bus_selector/21 -> PowertrainData_10_Ox176/1(in_port)  "<PowertrainData_10_Ox176>"
  bus_selector/22 -> PowertrainData_2_Ox42D/1(in_port)  "<PowertrainData_2_Ox42D>"
  bus_selector/23 -> PowertrainData_3_Ox43E/1(in_port)  "<PowertrainData_3_Ox43E>"
  bus_selector/24 -> PowertrainData_6_Ox205/1(in_port)  "<PowertrainData_6_Ox205>"
  bus_selector/25 -> PowertrainData_7_Ox41F/1(in_port)  "<PowertrainData_7_Ox41F>"
  bus_selector/26 -> PowertrainData_9_Ox44C/1(in_port)  "<PowertrainData_9_Ox44C>"
  bus_selector/27 -> Powertrain_Data_4_Ox424/1(in_port)  "<Powertrain_Data_4_Ox424>"
  bus_selector/28 -> Powertrain_Data_5_Ox43F/1(in_port)  "<Powertrain_Data_5_Ox43F>"
  bus_selector/29 -> Stop_Start_Ox166/1(in_port)  "<Stop_Start_Ox166>"
  bus_selector/30 -> TesterPhysicalResPCM_Ox7E8/1(in_port)  "<TesterPhysicalResPCM_Ox7E8>"
  bus_selector/31 -> TorqueDataEngFlags_Ox200/1(in_port)  "<TorqueDataEngFlags_Ox200>"
  bus_selector/32 -> TransGearData_Ox230/1(in_port)  "<TransGearData_Ox230>"
  bus_selector/33 -> VehicleOperatingModes_Ox167/1(in_port)  "<VehicleOperatingModes_Ox167>"

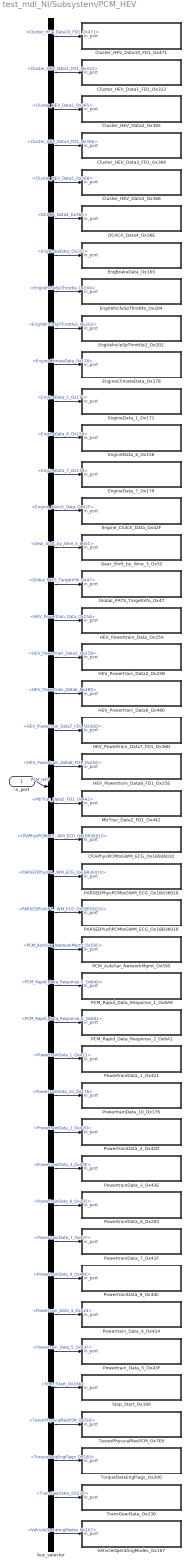
== system test_mdl_NI/Subsystem/PCM_HEV ==
  in_port : Inport
  Cluster_HEV_Data10_FD1_Ox471 : Subsystem
  Cluster_HEV_Data1_FD1_Ox312 : Subsystem
  Cluster_HEV_Data2_Ox365 : Subsystem
  Cluster_HEV_Data3_FD1_Ox366 : Subsystem
  Cluster_HEV_Data5_Ox368 : Subsystem
  DCACA_Data4_Ox36E : Subsystem
  EngBrakeData_Ox165 : Subsystem
  EngVehicleSpThrottle2_Ox202 : Subsystem
  EngVehicleSpThrottle_Ox204 : Subsystem
  EngineClimateData_Ox178 : Subsystem
  EngineData_1_Ox171 : Subsystem
  EngineData_6_Ox156 : Subsystem
  EngineData_7_Ox179 : Subsystem
  Engine_Clutch_Data_Ox42F : Subsystem
  Gear_Shift_by_Wire_3_Ox5C : Subsystem
  Global_PATS_TargetInfo_Ox47 : Subsystem
  HEV_Powertrain_Data2_Ox25B : Subsystem
  HEV_Powertrain_Data6_Ox480 : Subsystem
  HEV_Powertrain_Data7_FD1_Ox36D : Subsystem
  HEV_Powertrain_Data8_FD1_Ox25E : Subsystem
  HEV_Powertrain_Data_Ox25A : Subsystem
  MtrTrac_Data2_FD1_Ox442 : Subsystem
  OTAPhysPCMtoGWM_ECG_Ox1B936010 : Subsystem
  PARSEDPhysPCMtoGWM_ECG_Ox1BA36010 : Subsystem
  PARSEDPushPCMtoGWM_ECG_Ox1BB36010 : Subsystem
  PCM_AutoSar_NetworkMgmt_Ox595 : Subsystem
  PCM_Rapid_Data_Response_1_Ox6A0 : Subsystem
  PCM_Rapid_Data_Response_2_Ox6A1 : Subsystem
  PowertrainData_10_Ox176 : Subsystem
  PowertrainData_1_Ox421 : Subsystem
  PowertrainData_2_Ox42D : Subsystem
  PowertrainData_3_Ox43E : Subsystem
  PowertrainData_6_Ox205 : Subsystem
  PowertrainData_7_Ox41F : Subsystem
  PowertrainData_9_Ox44C : Subsystem
  Powertrain_Data_4_Ox424 : Subsystem
  Powertrain_Data_5_Ox43F : Subsystem
  Stop_Start_Ox166 : Subsystem
  TesterPhysicalResPCM_Ox7E8 : Subsystem
  TorqueDataEngFlags_Ox200 : Subsystem
  TransGearData_Ox230 : Subsystem
  VehicleOperatingModes_Ox167 : Subsystem
  bus_selector : BusSelector  OutputSignals=Cluster_HEV_Data10_FD1_Ox471,Cluster_HEV_Data1_FD1_Ox312,Cluster_HEV_Data2_Ox365,Cluster_HEV_Data3_FD1_Ox366,Cluster_HEV_Data5_Ox368,DCACA_Data4_Ox36E,EngBrakeData_Ox165,EngVehicleSpThrottle_Ox204,EngVehicleSpThrottle2_Ox202,EngineClimateData_Ox178,EngineData_1_Ox171,EngineData_6_Ox156,EngineData_7_Ox179,Engine_Clutch_Data_Ox42F,Gear_Shift_by_Wire_3_Ox5C,Global_PATS_TargetInfo_Ox47,HEV_Powertrain_Data_Ox25A,HEV_Powertrain_Data2_Ox25B,HEV_Powertrain_Data6_Ox480,HEV_Powertrain_Data7_FD1_Ox36D,HEV_Powertrain_Data8_FD1_Ox25E,MtrTrac_Data2_FD1_Ox442,OTAPhysPCMtoGWM_ECG_Ox1B936010,PARSEDPhysPCMtoGWM_ECG_Ox1BA36010,PARSEDPushPCMtoGWM_ECG_Ox1BB36010,PCM_AutoSar_NetworkMgmt_Ox595,PCM_Rapid_Data_Response_1_Ox6A0,PCM_Rapid_Data_Response_2_Ox6A1,PowertrainData_1_Ox421,PowertrainData_10_Ox176,PowertrainData_2_Ox42D,PowertrainData_3_Ox43E,PowertrainData_6_Ox205,PowertrainData_7_Ox41F,PowertrainData_9_Ox44C,Powertrain_Data_4_Ox424,Powertrain_Data_5_Ox43F,Stop_Start_Ox166,TesterPhysicalResPCM_Ox7E8,TorqueDataEngFlags_Ox200,TransGearData_Ox230,VehicleOperatingModes_Ox167
  wires:
  in_port/1 -> bus_selector/1  "PCM_HEV"
  bus_selector/1 -> Cluster_HEV_Data10_FD1_Ox471/1(in_port)  "<Cluster_HEV_Data10_FD1_Ox471>"
  bus_selector/2 -> Cluster_HEV_Data1_FD1_Ox312/1(in_port)  "<Cluster_HEV_Data1_FD1_Ox312>"
  bus_selector/3 -> Cluster_HEV_Data2_Ox365/1(in_port)  "<Cluster_HEV_Data2_Ox365>"
  bus_selector/4 -> Cluster_HEV_Data3_FD1_Ox366/1(in_port)  "<Cluster_HEV_Data3_FD1_Ox366>"
  bus_selector/5 -> Cluster_HEV_Data5_Ox368/1(in_port)  "<Cluster_HEV_Data5_Ox368>"
  bus_selector/6 -> DCACA_Data4_Ox36E/1(in_port)  "<DCACA_Data4_Ox36E>"
  bus_selector/7 -> EngBrakeData_Ox165/1(in_port)  "<EngBrakeData_Ox165>"
  bus_selector/8 -> EngVehicleSpThrottle_Ox204/1(in_port)  "<EngVehicleSpThrottle_Ox204>"
  bus_selector/9 -> EngVehicleSpThrottle2_Ox202/1(in_port)  "<EngVehicleSpThrottle2_Ox202>"
  bus_selector/10 -> EngineClimateData_Ox178/1(in_port)  "<EngineClimateData_Ox178>"
  bus_selector/11 -> EngineData_1_Ox171/1(in_port)  "<EngineData_1_Ox171>"
  bus_selector/12 -> EngineData_6_Ox156/1(in_port)  "<EngineData_6_Ox156>"
  bus_selector/13 -> EngineData_7_Ox179/1(in_port)  "<EngineData_7_Ox179>"
  bus_selector/14 -> Engine_Clutch_Data_Ox42F/1(in_port)  "<Engine_Clutch_Data_Ox42F>"
  bus_selector/15 -> Gear_Shift_by_Wire_3_Ox5C/1(in_port)  "<Gear_Shift_by_Wire_3_Ox5C>"
  bus_selector/16 -> Global_PATS_TargetInfo_Ox47/1(in_port)  "<Global_PATS_TargetInfo_Ox47>"
  bus_selector/17 -> HEV_Powertrain_Data_Ox25A/1(in_port)  "<HEV_Powertrain_Data_Ox25A>"
  bus_selector/18 -> HEV_Powertrain_Data2_Ox25B/1(in_port)  "<HEV_Powertrain_Data2_Ox25B>"
  bus_selector/19 -> HEV_Powertrain_Data6_Ox480/1(in_port)  "<HEV_Powertrain_Data6_Ox480>"
  bus_selector/20 -> HEV_Powertrain_Data7_FD1_Ox36D/1(in_port)  "<HEV_Powertrain_Data7_FD1_Ox36D>"
  bus_selector/21 -> HEV_Powertrain_Data8_FD1_Ox25E/1(in_port)  "<HEV_Powertrain_Data8_FD1_Ox25E>"
  bus_selector/22 -> MtrTrac_Data2_FD1_Ox442/1(in_port)  "<MtrTrac_Data2_FD1_Ox442>"
  bus_selector/23 -> OTAPhysPCMtoGWM_ECG_Ox1B936010/1(in_port)  "<OTAPhysPCMtoGWM_ECG_Ox1B936010>"
  bus_selector/24 -> PARSEDPhysPCMtoGWM_ECG_Ox1BA36010/1(in_port)  "<PARSEDPhysPCMtoGWM_ECG_Ox1BA36010>"
  bus_selector/25 -> PARSEDPushPCMtoGWM_ECG_Ox1BB36010/1(in_port)  "<PARSEDPushPCMtoGWM_ECG_Ox1BB36010>"
  bus_selector/26 -> PCM_AutoSar_NetworkMgmt_Ox595/1(in_port)  "<PCM_AutoSar_NetworkMgmt_Ox595>"
  bus_selector/27 -> PCM_Rapid_Data_Response_1_Ox6A0/1(in_port)  "<PCM_Rapid_Data_Response_1_Ox6A0>"
  bus_selector/28 -> PCM_Rapid_Data_Response_2_Ox6A1/1(in_port)  "<PCM_Rapid_Data_Response_2_Ox6A1>"
  bus_selector/29 -> PowertrainData_1_Ox421/1(in_port)  "<PowertrainData_1_Ox421>"
  bus_selector/30 -> PowertrainData_10_Ox176/1(in_port)  "<PowertrainData_10_Ox176>"
  bus_selector/31 -> PowertrainData_2_Ox42D/1(in_port)  "<PowertrainData_2_Ox42D>"
  bus_selector/32 -> PowertrainData_3_Ox43E/1(in_port)  "<PowertrainData_3_Ox43E>"
  bus_selector/33 -> PowertrainData_6_Ox205/1(in_port)  "<PowertrainData_6_Ox205>"
  bus_selector/34 -> PowertrainData_7_Ox41F/1(in_port)  "<PowertrainData_7_Ox41F>"
  bus_selector/35 -> PowertrainData_9_Ox44C/1(in_port)  "<PowertrainData_9_Ox44C>"
  bus_selector/36 -> Powertrain_Data_4_Ox424/1(in_port)  "<Powertrain_Data_4_Ox424>"
  bus_selector/37 -> Powertrain_Data_5_Ox43F/1(in_port)  "<Powertrain_Data_5_Ox43F>"
  bus_selector/38 -> Stop_Start_Ox166/1(in_port)  "<Stop_Start_Ox166>"
  bus_selector/39 -> TesterPhysicalResPCM_Ox7E8/1(in_port)  "<TesterPhysicalResPCM_Ox7E8>"
  bus_selector/40 -> TorqueDataEngFlags_Ox200/1(in_port)  "<TorqueDataEngFlags_Ox200>"
  bus_selector/41 -> TransGearData_Ox230/1(in_port)  "<TransGearData_Ox230>"
  bus_selector/42 -> VehicleOperatingModes_Ox167/1(in_port)  "<VehicleOperatingModes_Ox167>"

== system test_mdl_NI/Subsystem/PSCM ==
  in_port : Inport
  EPAS_INFO_Ox82 : Subsystem
  Lane_Assist_Data3_FD1_Ox3CC : Subsystem
  PSCM_AutoSar_NetwrkMgmt_Ox5B5 : Subsystem
  SteeringPinion_Data_Ox7E : Subsystem
  TesterPhysicalResPSCM_Ox738 : Subsystem
  TrailerAid_Data2_Ox417 : Subsystem
  bus_selector : BusSelector  OutputSignals=EPAS_INFO_Ox82,Lane_Assist_Data3_FD1_Ox3CC,PSCM_AutoSar_NetwrkMgmt_Ox5B5,SteeringPinion_Data_Ox7E,TesterPhysicalResPSCM_Ox738,TrailerAid_Data2_Ox417
  wires:
  in_port/1 -> bus_selector/1  "PSCM"
  bus_selector/1 -> EPAS_INFO_Ox82/1(in_port)  "<EPAS_INFO_Ox82>"
  bus_selector/2 -> Lane_Assist_Data3_FD1_Ox3CC/1(in_port)  "<Lane_Assist_Data3_FD1_Ox3CC>"
  bus_selector/3 -> PSCM_AutoSar_NetwrkMgmt_Ox5B5/1(in_port)  "<PSCM_AutoSar_NetwrkMgmt_Ox5B5>"
  bus_selector/4 -> SteeringPinion_Data_Ox7E/1(in_port)  "<SteeringPinion_Data_Ox7E>"
  bus_selector/5 -> TesterPhysicalResPSCM_Ox738/1(in_port)  "<TesterPhysicalResPSCM_Ox738>"
  bus_selector/6 -> TrailerAid_Data2_Ox417/1(in_port)  "<TrailerAid_Data2_Ox417>"

== system test_mdl_NI/Subsystem/SOBDMC_HPCM_FD1 ==
  in_port : Inport
  AC_Compressor_Req_FD1_Ox410 : Subsystem
  ChargeSettings_FD1_Ox3F5 : Subsystem
  Cluster_HEV_Data1_FD1_Ox312 : Subsystem
  Cluster_HEV_Data4_FD1_Ox367 : Subsystem
  Cluster_HEV_Data5_Ox368 : Subsystem
  Cluster_HEV_Data7_FD1_Ox474 : Subsystem
  Cluster_HEV_Data9_FD1_Ox475 : Subsystem
  ConsTip_Data_FD1_Ox476 : Subsystem
  GWM_HPCM_i_FrP10_FD1_Ox472 : Subsystem
  GWM_HPCM_i_FrP11_FD1_Ox473 : Subsystem
  Global_PATS_Target2_FD1_Ox48 : Subsystem
  GoTimeSettings_FD1_Ox3F8 : Subsystem
  HEV_ChargeStat_FD1_Ox352 : Subsystem
  MHT_EV_Wakeup_FD1_Ox478 : Subsystem
  MtrTracData_1_FD1_Ox441 : Subsystem
  MtrTrac_Data2_FD1_Ox442 : Subsystem
  OTAPhysSOBDMCtoGWM_FD1_Ox1B936011 : Subsystem
  PARSEDHPCMtoGWM_ECG_FD1_Ox1BA36011 : Subsystem
  PARSEDPushSOBDMCtoGWM_FD1_Ox1BB36011 : Subsystem
  PreCond_Hev_Data1_FD1_Ox440 : Subsystem
  PreCond_Hev_Data2_FD1_Ox185 : Subsystem
  SOBDMC_AutoSar_NetMgmt_FD1_Ox5A5 : Subsystem
  SOBDMC_RapidData_Resp1_FD1_Ox68C : Subsystem
  SOBDMC_RapidData_Resp2_FD1_Ox68D : Subsystem
  SOBDMC_RapidData_Resp3_FD1_Ox68E : Subsystem
  SOBDMC_RapidData_Resp4_FD1_Ox68F : Subsystem
  Saved_Charge_Location_FD1_Ox3F4 : Subsystem
  TesterPhysicalResSOBDMCFD1_Ox7EE : Subsystem
  Unsaved_Charge_LocationFD1_Ox3F3 : Subsystem
  bus_selector : BusSelector  OutputSignals=AC_Compressor_Req_FD1_Ox410,ChargeSettings_FD1_Ox3F5,Cluster_HEV_Data1_FD1_Ox312,Cluster_HEV_Data4_FD1_Ox367,Cluster_HEV_Data5_Ox368,Cluster_HEV_Data7_FD1_Ox474,Cluster_HEV_Data9_FD1_Ox475,ConsTip_Data_FD1_Ox476,GWM_HPCM_i_FrP10_FD1_Ox472,GWM_HPCM_i_FrP11_FD1_Ox473,Global_PATS_Target2_FD1_Ox48,GoTimeSettings_FD1_Ox3F8,HEV_ChargeStat_FD1_Ox352,MHT_EV_Wakeup_FD1_Ox478,MtrTracData_1_FD1_Ox441,MtrTrac_Data2_FD1_Ox442,OTAPhysSOBDMCtoGWM_FD1_Ox1B936011,PARSEDHPCMtoGWM_ECG_FD1_Ox1BA36011,PARSEDPushSOBDMCtoGWM_FD1_Ox1BB36011,PreCond_Hev_Data1_FD1_Ox440,PreCond_Hev_Data2_FD1_Ox185,SOBDMC_AutoSar_NetMgmt_FD1_Ox5A5,SOBDMC_RapidData_Resp1_FD1_Ox68C,SOBDMC_RapidData_Resp2_FD1_Ox68D,SOBDMC_RapidData_Resp3_FD1_Ox68E,SOBDMC_RapidData_Resp4_FD1_Ox68F,Saved_Charge_Location_FD1_Ox3F4,TesterPhysicalResSOBDMCFD1_Ox7EE,Unsaved_Charge_LocationFD1_Ox3F3
  wires:
  in_port/1 -> bus_selector/1  "SOBDMC_HPCM_FD1"
  bus_selector/1 -> AC_Compressor_Req_FD1_Ox410/1(in_port)  "<AC_Compressor_Req_FD1_Ox410>"
  bus_selector/2 -> ChargeSettings_FD1_Ox3F5/1(in_port)  "<ChargeSettings_FD1_Ox3F5>"
  bus_selector/3 -> Cluster_HEV_Data1_FD1_Ox312/1(in_port)  "<Cluster_HEV_Data1_FD1_Ox312>"
  bus_selector/4 -> Cluster_HEV_Data4_FD1_Ox367/1(in_port)  "<Cluster_HEV_Data4_FD1_Ox367>"
  bus_selector/5 -> Cluster_HEV_Data5_Ox368/1(in_port)  "<Cluster_HEV_Data5_Ox368>"
  bus_selector/6 -> Cluster_HEV_Data7_FD1_Ox474/1(in_port)  "<Cluster_HEV_Data7_FD1_Ox474>"
  bus_selector/7 -> Cluster_HEV_Data9_FD1_Ox475/1(in_port)  "<Cluster_HEV_Data9_FD1_Ox475>"
  bus_selector/8 -> ConsTip_Data_FD1_Ox476/1(in_port)  "<ConsTip_Data_FD1_Ox476>"
  bus_selector/9 -> GWM_HPCM_i_FrP10_FD1_Ox472/1(in_port)  "<GWM_HPCM_i_FrP10_FD1_Ox472>"
  bus_selector/10 -> GWM_HPCM_i_FrP11_FD1_Ox473/1(in_port)  "<GWM_HPCM_i_FrP11_FD1_Ox473>"
  bus_selector/11 -> Global_PATS_Target2_FD1_Ox48/1(in_port)  "<Global_PATS_Target2_FD1_Ox48>"
  bus_selector/12 -> GoTimeSettings_FD1_Ox3F8/1(in_port)  "<GoTimeSettings_FD1_Ox3F8>"
  bus_selector/13 -> HEV_ChargeStat_FD1_Ox352/1(in_port)  "<HEV_ChargeStat_FD1_Ox352>"
  bus_selector/14 -> MHT_EV_Wakeup_FD1_Ox478/1(in_port)  "<MHT_EV_Wakeup_FD1_Ox478>"
  bus_selector/15 -> MtrTracData_1_FD1_Ox441/1(in_port)  "<MtrTracData_1_FD1_Ox441>"
  bus_selector/16 -> MtrTrac_Data2_FD1_Ox442/1(in_port)  "<MtrTrac_Data2_FD1_Ox442>"
  bus_selector/17 -> OTAPhysSOBDMCtoGWM_FD1_Ox1B936011/1(in_port)  "<OTAPhysSOBDMCtoGWM_FD1_Ox1B936011>"
  bus_selector/18 -> PARSEDHPCMtoGWM_ECG_FD1_Ox1BA36011/1(in_port)  "<PARSEDHPCMtoGWM_ECG_FD1_Ox1BA36011>"
  bus_selector/19 -> PARSEDPushSOBDMCtoGWM_FD1_Ox1BB36011/1(in_port)  "<PARSEDPushSOBDMCtoGWM_FD1_Ox1BB36011>"
  bus_selector/20 -> PreCond_Hev_Data1_FD1_Ox440/1(in_port)  "<PreCond_Hev_Data1_FD1_Ox440>"
  bus_selector/21 -> PreCond_Hev_Data2_FD1_Ox185/1(in_port)  "<PreCond_Hev_Data2_FD1_Ox185>"
  bus_selector/22 -> SOBDMC_AutoSar_NetMgmt_FD1_Ox5A5/1(in_port)  "<SOBDMC_AutoSar_NetMgmt_FD1_Ox5A5>"
  bus_selector/23 -> SOBDMC_RapidData_Resp1_FD1_Ox68C/1(in_port)  "<SOBDMC_RapidData_Resp1_FD1_Ox68C>"
  bus_selector/24 -> SOBDMC_RapidData_Resp2_FD1_Ox68D/1(in_port)  "<SOBDMC_RapidData_Resp2_FD1_Ox68D>"
  bus_selector/25 -> SOBDMC_RapidData_Resp3_FD1_Ox68E/1(in_port)  "<SOBDMC_RapidData_Resp3_FD1_Ox68E>"
  bus_selector/26 -> SOBDMC_RapidData_Resp4_FD1_Ox68F/1(in_port)  "<SOBDMC_RapidData_Resp4_FD1_Ox68F>"
  bus_selector/27 -> Saved_Charge_Location_FD1_Ox3F4/1(in_port)  "<Saved_Charge_Location_FD1_Ox3F4>"
  bus_selector/28 -> TesterPhysicalResSOBDMCFD1_Ox7EE/1(in_port)  "<TesterPhysicalResSOBDMCFD1_Ox7EE>"
  bus_selector/29 -> Unsaved_Charge_LocationFD1_Ox3F3/1(in_port)  "<Unsaved_Charge_LocationFD1_Ox3F3>"

== system test_mdl_NI/Subsystem/TCCM ==
  in_port : Inport
  AWD_Torque_Data_Ox20C : Subsystem
  Driveline_Data_1_Ox263 : Subsystem
  Driveline_Data_2_Ox4A2 : Subsystem
  TCCM_AutoSar_NetwkMgmt_Ox5A1 : Subsystem
  TesterPhysicalResTCCM_Ox769 : Subsystem
  bus_selector : BusSelector  OutputSignals=AWD_Torque_Data_Ox20C,Driveline_Data_1_Ox263,Driveline_Data_2_Ox4A2,TCCM_AutoSar_NetwkMgmt_Ox5A1,TesterPhysicalResTCCM_Ox769
  wires:
  in_port/1 -> bus_selector/1  "TCCM"
  bus_selector/1 -> AWD_Torque_Data_Ox20C/1(in_port)  "<AWD_Torque_Data_Ox20C>"
  bus_selector/2 -> Driveline_Data_1_Ox263/1(in_port)  "<Driveline_Data_1_Ox263>"
  bus_selector/3 -> Driveline_Data_2_Ox4A2/1(in_port)  "<Driveline_Data_2_Ox4A2>"
  bus_selector/4 -> TCCM_AutoSar_NetwkMgmt_Ox5A1/1(in_port)  "<TCCM_AutoSar_NetwkMgmt_Ox5A1>"
  bus_selector/5 -> TesterPhysicalResTCCM_Ox769/1(in_port)  "<TesterPhysicalResTCCM_Ox769>"

== system test_mdl_NI/Subsystem/TCM_DSL ==
  in_port : Inport
  EngineData_1_Ox171 : Subsystem
  Gear_Shift_by_Wire_3_Ox5C : Subsystem
  PowertrainData_10_Ox176 : Subsystem
  TCM_AutoSar_NetworkMgt_Ox5A0 : Subsystem
  TCM_Rapid_Data_Response_1_Ox6A4 : Subsystem
  TCM_Rapid_Data_Response_2_Ox6A5 : Subsystem
  TesterPhysicalResTCM_Ox7E9 : Subsystem
  TransData_3_Ox14A : Subsystem
  TransGearData_2_Ox231 : Subsystem
  TransGearData_Ox230 : Subsystem
  bus_selector : BusSelector  OutputSignals=EngineData_1_Ox171,Gear_Shift_by_Wire_3_Ox5C,PowertrainData_10_Ox176,TCM_AutoSar_NetworkMgt_Ox5A0,TCM_Rapid_Data_Response_1_Ox6A4,TCM_Rapid_Data_Response_2_Ox6A5,TesterPhysicalResTCM_Ox7E9,TransData_3_Ox14A,TransGearData_Ox230,TransGearData_2_Ox231
  wires:
  in_port/1 -> bus_selector/1  "TCM_DSL"
  bus_selector/1 -> EngineData_1_Ox171/1(in_port)  "<EngineData_1_Ox171>"
  bus_selector/2 -> Gear_Shift_by_Wire_3_Ox5C/1(in_port)  "<Gear_Shift_by_Wire_3_Ox5C>"
  bus_selector/3 -> PowertrainData_10_Ox176/1(in_port)  "<PowertrainData_10_Ox176>"
  bus_selector/4 -> TCM_AutoSar_NetworkMgt_Ox5A0/1(in_port)  "<TCM_AutoSar_NetworkMgt_Ox5A0>"
  bus_selector/5 -> TCM_Rapid_Data_Response_1_Ox6A4/1(in_port)  "<TCM_Rapid_Data_Response_1_Ox6A4>"
  bus_selector/6 -> TCM_Rapid_Data_Response_2_Ox6A5/1(in_port)  "<TCM_Rapid_Data_Response_2_Ox6A5>"
  bus_selector/7 -> TesterPhysicalResTCM_Ox7E9/1(in_port)  "<TesterPhysicalResTCM_Ox7E9>"
  bus_selector/8 -> TransData_3_Ox14A/1(in_port)  "<TransData_3_Ox14A>"
  bus_selector/9 -> TransGearData_Ox230/1(in_port)  "<TransGearData_Ox230>"
  bus_selector/10 -> TransGearData_2_Ox231/1(in_port)  "<TransGearData_2_Ox231>"

== system test_mdl_NI/Subsystem/TSTR ==
  in_port : Inport
  TesterFunctionalReq_FD1_Ox7DF : Subsystem
  TesterPhysicalReqABS_Ox760 : Subsystem
  TesterPhysicalReqCCM_Ox764 : Subsystem
  TesterPhysicalReqCMR_DSMC_Ox7C1 : Subsystem
  TesterPhysicalReqGWM_FD1_Ox716 : Subsystem
  TesterPhysicalReqIPMA_Ox706 : Subsystem
  TesterPhysicalReqPCM_Ox7E0 : Subsystem
  TesterPhysicalReqPSCM_Ox730 : Subsystem
  TesterPhysicalReqSOBDMC_FD_Ox7E6 : Subsystem
  TesterPhysicalReqSODCMC_Ox6F2 : Subsystem
  TesterPhysicalReqSODCMD_Ox6F3 : Subsystem
  TesterPhysicalReqSODL_Ox7C4 : Subsystem
  TesterPhysicalReqSODR_Ox7C6 : Subsystem
  TesterPhysicalReqTCCM_Ox761 : Subsystem
  TesterPhysicalReqTCM_Ox7E1 : Subsystem
  bus_selector : BusSelector  OutputSignals=TesterFunctionalReq_FD1_Ox7DF,TesterPhysicalReqABS_Ox760,TesterPhysicalReqCCM_Ox764,TesterPhysicalReqCMR_DSMC_Ox7C1,TesterPhysicalReqGWM_FD1_Ox716,TesterPhysicalReqIPMA_Ox706,TesterPhysicalReqPCM_Ox7E0,TesterPhysicalReqPSCM_Ox730,TesterPhysicalReqSOBDMC_FD_Ox7E6,TesterPhysicalReqSODCMC_Ox6F2,TesterPhysicalReqSODCMD_Ox6F3,TesterPhysicalReqSODL_Ox7C4,TesterPhysicalReqSODR_Ox7C6,TesterPhysicalReqTCCM_Ox761,TesterPhysicalReqTCM_Ox7E1
  wires:
  in_port/1 -> bus_selector/1  "TSTR"
  bus_selector/1 -> TesterFunctionalReq_FD1_Ox7DF/1(in_port)  "<TesterFunctionalReq_FD1_Ox7DF>"
  bus_selector/2 -> TesterPhysicalReqABS_Ox760/1(in_port)  "<TesterPhysicalReqABS_Ox760>"
  bus_selector/3 -> TesterPhysicalReqCCM_Ox764/1(in_port)  "<TesterPhysicalReqCCM_Ox764>"
  bus_selector/4 -> TesterPhysicalReqCMR_DSMC_Ox7C1/1(in_port)  "<TesterPhysicalReqCMR_DSMC_Ox7C1>"
  bus_selector/5 -> TesterPhysicalReqGWM_FD1_Ox716/1(in_port)  "<TesterPhysicalReqGWM_FD1_Ox716>"
  bus_selector/6 -> TesterPhysicalReqIPMA_Ox706/1(in_port)  "<TesterPhysicalReqIPMA_Ox706>"
  bus_selector/7 -> TesterPhysicalReqPCM_Ox7E0/1(in_port)  "<TesterPhysicalReqPCM_Ox7E0>"
  bus_selector/8 -> TesterPhysicalReqPSCM_Ox730/1(in_port)  "<TesterPhysicalReqPSCM_Ox730>"
  bus_selector/9 -> TesterPhysicalReqSOBDMC_FD_Ox7E6/1(in_port)  "<TesterPhysicalReqSOBDMC_FD_Ox7E6>"
  bus_selector/10 -> TesterPhysicalReqSODCMC_Ox6F2/1(in_port)  "<TesterPhysicalReqSODCMC_Ox6F2>"
  bus_selector/11 -> TesterPhysicalReqSODCMD_Ox6F3/1(in_port)  "<TesterPhysicalReqSODCMD_Ox6F3>"
  bus_selector/12 -> TesterPhysicalReqSODL_Ox7C4/1(in_port)  "<TesterPhysicalReqSODL_Ox7C4>"
  bus_selector/13 -> TesterPhysicalReqSODR_Ox7C6/1(in_port)  "<TesterPhysicalReqSODR_Ox7C6>"
  bus_selector/14 -> TesterPhysicalReqTCCM_Ox761/1(in_port)  "<TesterPhysicalReqTCCM_Ox761>"
  bus_selector/15 -> TesterPhysicalReqTCM_Ox7E1/1(in_port)  "<TesterPhysicalReqTCM_Ox7E1>"

== system test_mdl_NI/Subsystem/VDM ==
  in_port : Inport
  Suspension_Data_Ox23A : Subsystem
  TesterPhysicalResVDM_Ox729 : Subsystem
  VeyDynamics_Data_Ox345 : Subsystem
  bus_selector : BusSelector  OutputSignals=Suspension_Data_Ox23A,TesterPhysicalResVDM_Ox729,VeyDynamics_Data_Ox345
  wires:
  in_port/1 -> bus_selector/1  "VDM"
  bus_selector/1 -> Suspension_Data_Ox23A/1(in_port)  "<Suspension_Data_Ox23A>"
  bus_selector/2 -> TesterPhysicalResVDM_Ox729/1(in_port)  "<TesterPhysicalResVDM_Ox729>"
  bus_selector/3 -> VeyDynamics_Data_Ox345/1(in_port)  "<VeyDynamics_Data_Ox345>"

== system test_mdl_NI/To_NI_HIL/DSMC ==
  in : Inport
  DrvStatMonData : Subsystem
  bus_creator : BusCreator  Inputs=1
  bus_selector : BusSelector  OutputSignals=DrvStatMonData
  out_port : Outport
  wires:
  bus_creator/1 -> out_port/1  "DSMC"
  DrvStatMonData/1(out_port) -> bus_creator/1  "DrvStatMonData"
  bus_selector/1 -> DrvStatMonData/1(in)  "<DrvStatMonData>"
  in/1 -> bus_selector/1
